simulink model "FinalSim"  (R2022b)
settings: Solver=VariableStepAuto  StartTime=0.0  StopTime=10  RelTol=1e-3
libraries: eeGeneralControl x3
(part 6 of 7)

== system FinalSim/Bicep Model/Bicep Group1/fascicles (CE & PE)/Type F Motor Units/Motor Unit 1 ==
  fenv : Inport
  Y,L : Inport  Port=2
  1/Tf (feff' < 0) : Fcn  Expr=u(2)/(0.02822+0.01513*u(3))
  1/Tf (feff' > 0) : Fcn  Expr=1/(0.02057*u(2)^2+0.0136*u(4))
  1/Ts : Gain  Gain=23.2558  SaturateOnIntegerOverflow=on  OutDataTypeStr=Inherit: Same as input  ParamDataTypeStr=Inherit: Same as input
  Af : Fcn  Expr=1-exp(-(u(1)*u(4)*u(3)/(0.56*u(2)))^u(2))
  Leff' : Fcn  Expr=(u(2)-u(1))^3/((1-u(3))*8.8e-005)
  Leff'->Leff : Integrator  InitialCondition=1
  "Leff,L, Af,fenv" : Mux
  S and old S diff : Sum  Inputs=-+  InputSameDT=on  SaturateOnIntegerOverflow=on  OutDataTypeStr=Inherit: Same as first input
  Y,nf,feff,S : Mux
  aS1 : Constant  Value=1.76
  aS2 : Constant  Value=0.96
  demux Y,L : Demux  Outputs=2
      settings: DisplayOption=none
  feff' : Product  InputSameDT=on  RndMeth=Zero  SaturateOnIntegerOverflow=on  OutDataTypeStr=Inherit: Same as first input
  feff' > 0? : Switch
  feff'->feff : Integrator
  feff>0.1? : Switch  Threshold=0.1
  fenv-fint : Sum  Inputs=+-  InputSameDT=on  SaturateOnIntegerOverflow=on  OutDataTypeStr=Inherit: Same as first input
  fint' : Product  InputSameDT=on  RndMeth=Zero  SaturateOnIntegerOverflow=on  OutDataTypeStr=Inherit: Same as first input
  fint'->fint : Integrator
  fint-feff : Sum  Inputs=+-  InputSameDT=on  SaturateOnIntegerOverflow=on  OutDataTypeStr=Inherit: Same as first input
  nf : Fcn  Expr=2.11+3.31*(1/u-1)
  s'->s : Integrator  InitialCondition=1.76
  A : Outport
  wires:
  Y,L/1 -> demux Y,L/1
  demux Y,L/1 -> Y,nf,feff,S/1
  demux Y,L/2 -> "Leff,L, Af,fenv"/2
  "Leff,L, Af,fenv"/1 -> 1/Tf (feff' < 0)/1, Leff'/1, 1/Tf (feff' > 0)/1
  1/Tf (feff' > 0)/1 -> feff' > 0?/1
  1/Tf (feff' < 0)/1 -> feff' > 0?/3
  fenv/1 -> fenv-fint/1, "Leff,L, Af,fenv"/4
  fenv-fint/1 -> fint'/2
  fint'/1 -> fint'->fint/1
  fint'->fint/1 -> fint-feff/1, fenv-fint/2
  fint-feff/1 -> feff'/2, feff' > 0?/2
  feff' > 0?/1 -> feff'/1, fint'/1
  feff'/1 -> feff'->feff/1
  feff'->feff/1 -> fint-feff/2, Y,nf,feff,S/3, feff>0.1?/2
  Y,nf,feff,S/1 -> Af/1
  Af/1 -> "Leff,L, Af,fenv"/3, A/1
  Leff'/1 -> Leff'->Leff/1
  Leff'->Leff/1 -> "Leff,L, Af,fenv"/1, nf/1
  nf/1 -> Y,nf,feff,S/2
  aS2/1 -> feff>0.1?/1
  aS1/1 -> feff>0.1?/3
  feff>0.1?/1 -> S and old S diff/2
  S and old S diff/1 -> 1/Ts/1
  1/Ts/1 -> s'->s/1
  s'->s/1 -> S and old S diff/1, Y,nf,feff,S/4

== system FinalSim/Bicep Model/Bicep Group1/fascicles (CE & PE)/Type F Motor Units/Motor Unit 2 ==
  fenv : Inport
  Y,L : Inport  Port=2
  1/Tf (feff' < 0) : Fcn  Expr=u(2)/(0.02822+0.01513*u(3))
  1/Tf (feff' > 0) : Fcn  Expr=1/(0.02057*u(2)^2+0.0136*u(4))
  1/Ts : Gain  Gain=23.2558  SaturateOnIntegerOverflow=on  OutDataTypeStr=Inherit: Same as input  ParamDataTypeStr=Inherit: Same as input
  Af : Fcn  Expr=1-exp(-(u(1)*u(4)*u(3)/(0.56*u(2)))^u(2))
  Leff' : Fcn  Expr=(u(2)-u(1))^3/((1-u(3))*8.8e-005)
  Leff'->Leff : Integrator  InitialCondition=1
  "Leff,L, Af,fenv" : Mux
  S and old S diff : Sum  Inputs=-+  InputSameDT=on  SaturateOnIntegerOverflow=on  OutDataTypeStr=Inherit: Same as first input
  Y,nf,feff,S : Mux
  aS1 : Constant  Value=1.76
  aS2 : Constant  Value=0.96
  demux Y,L : Demux  Outputs=2
      settings: DisplayOption=none
  feff' : Product  InputSameDT=on  RndMeth=Zero  SaturateOnIntegerOverflow=on  OutDataTypeStr=Inherit: Same as first input
  feff' > 0? : Switch
  feff'->feff : Integrator
  feff>0.1? : Switch  Threshold=0.1
  fenv-fint : Sum  Inputs=+-  InputSameDT=on  SaturateOnIntegerOverflow=on  OutDataTypeStr=Inherit: Same as first input
  fint' : Product  InputSameDT=on  RndMeth=Zero  SaturateOnIntegerOverflow=on  OutDataTypeStr=Inherit: Same as first input
  fint'->fint : Integrator
  fint-feff : Sum  Inputs=+-  InputSameDT=on  SaturateOnIntegerOverflow=on  OutDataTypeStr=Inherit: Same as first input
  nf : Fcn  Expr=2.11+3.31*(1/u-1)
  s'->s : Integrator  InitialCondition=1.76
  A : Outport
  wires:
  Y,L/1 -> demux Y,L/1
  demux Y,L/1 -> Y,nf,feff,S/1
  demux Y,L/2 -> "Leff,L, Af,fenv"/2
  "Leff,L, Af,fenv"/1 -> 1/Tf (feff' < 0)/1, Leff'/1, 1/Tf (feff' > 0)/1
  1/Tf (feff' > 0)/1 -> feff' > 0?/1
  1/Tf (feff' < 0)/1 -> feff' > 0?/3
  fenv/1 -> fenv-fint/1, "Leff,L, Af,fenv"/4
  fenv-fint/1 -> fint'/2
  fint'/1 -> fint'->fint/1
  fint'->fint/1 -> fint-feff/1, fenv-fint/2
  fint-feff/1 -> feff'/2, feff' > 0?/2
  feff' > 0?/1 -> feff'/1, fint'/1
  feff'/1 -> feff'->feff/1
  feff'->feff/1 -> fint-feff/2, Y,nf,feff,S/3, feff>0.1?/2
  Y,nf,feff,S/1 -> Af/1
  Af/1 -> "Leff,L, Af,fenv"/3, A/1
  Leff'/1 -> Leff'->Leff/1
  Leff'->Leff/1 -> "Leff,L, Af,fenv"/1, nf/1
  nf/1 -> Y,nf,feff,S/2
  aS2/1 -> feff>0.1?/1
  aS1/1 -> feff>0.1?/3
  feff>0.1?/1 -> S and old S diff/2
  S and old S diff/1 -> 1/Ts/1
  1/Ts/1 -> s'->s/1
  s'->s/1 -> S and old S diff/1, Y,nf,feff,S/4

== system FinalSim/Bicep Model/Bicep Group1/fascicles (CE & PE)/Type F Motor Units/Motor Unit 3 ==
  fenv : Inport
  Y,L : Inport  Port=2
  1/Tf (feff' < 0) : Fcn  Expr=u(2)/(0.02822+0.01513*u(3))
  1/Tf (feff' > 0) : Fcn  Expr=1/(0.02057*u(2)^2+0.0136*u(4))
  1/Ts : Gain  Gain=23.2558  SaturateOnIntegerOverflow=on  OutDataTypeStr=Inherit: Same as input  ParamDataTypeStr=Inherit: Same as input
  Af : Fcn  Expr=1-exp(-(u(1)*u(4)*u(3)/(0.56*u(2)))^u(2))
  Leff' : Fcn  Expr=(u(2)-u(1))^3/((1-u(3))*8.8e-005)
  Leff'->Leff : Integrator  InitialCondition=1
  "Leff,L, Af,fenv" : Mux
  S and old S diff : Sum  Inputs=-+  InputSameDT=on  SaturateOnIntegerOverflow=on  OutDataTypeStr=Inherit: Same as first input
  Y,nf,feff,S : Mux
  aS1 : Constant  Value=1.76
  aS2 : Constant  Value=0.96
  demux Y,L : Demux  Outputs=2
      settings: DisplayOption=none
  feff' : Product  InputSameDT=on  RndMeth=Zero  SaturateOnIntegerOverflow=on  OutDataTypeStr=Inherit: Same as first input
  feff' > 0? : Switch
  feff'->feff : Integrator
  feff>0.1? : Switch  Threshold=0.1
  fenv-fint : Sum  Inputs=+-  InputSameDT=on  SaturateOnIntegerOverflow=on  OutDataTypeStr=Inherit: Same as first input
  fint' : Product  InputSameDT=on  RndMeth=Zero  SaturateOnIntegerOverflow=on  OutDataTypeStr=Inherit: Same as first input
  fint'->fint : Integrator
  fint-feff : Sum  Inputs=+-  InputSameDT=on  SaturateOnIntegerOverflow=on  OutDataTypeStr=Inherit: Same as first input
  nf : Fcn  Expr=2.11+3.31*(1/u-1)
  s'->s : Integrator  InitialCondition=1.76
  A : Outport
  wires:
  Y,L/1 -> demux Y,L/1
  demux Y,L/1 -> Y,nf,feff,S/1
  demux Y,L/2 -> "Leff,L, Af,fenv"/2
  "Leff,L, Af,fenv"/1 -> 1/Tf (feff' < 0)/1, Leff'/1, 1/Tf (feff' > 0)/1
  1/Tf (feff' > 0)/1 -> feff' > 0?/1
  1/Tf (feff' < 0)/1 -> feff' > 0?/3
  fenv/1 -> fenv-fint/1, "Leff,L, Af,fenv"/4
  fenv-fint/1 -> fint'/2
  fint'/1 -> fint'->fint/1
  fint'->fint/1 -> fint-feff/1, fenv-fint/2
  fint-feff/1 -> feff'/2, feff' > 0?/2
  feff' > 0?/1 -> feff'/1, fint'/1
  feff'/1 -> feff'->feff/1
  feff'->feff/1 -> fint-feff/2, Y,nf,feff,S/3, feff>0.1?/2
  Y,nf,feff,S/1 -> Af/1
  Af/1 -> "Leff,L, Af,fenv"/3, A/1
  Leff'/1 -> Leff'->Leff/1
  Leff'->Leff/1 -> "Leff,L, Af,fenv"/1, nf/1
  nf/1 -> Y,nf,feff,S/2
  aS2/1 -> feff>0.1?/1
  aS1/1 -> feff>0.1?/3
  feff>0.1?/1 -> S and old S diff/2
  S and old S diff/1 -> 1/Ts/1
  1/Ts/1 -> s'->s/1
  s'->s/1 -> S and old S diff/1, Y,nf,feff,S/4

== system FinalSim/Bicep Model/Bicep Group1/fascicles (CE & PE)/Type S Motor Units/Motor Unit 1 ==
  fenv : Inport
  Y,L : Inport  Port=2
  1/Tf (feff' < 0) : Fcn  Expr=u(2)/(0.047033+0.025217*u(3))
  1/Tf (feff' > 0) : Fcn  Expr=1/(0.034283*u(2)^2+0.022667*u(4))
  Af : Fcn  Expr=1-exp(-(u(1)*u(4)*u(3)/(0.56*u(2)))^u(2))
  Leff' : Fcn  Expr=(u(2)-u(1))^3/((1-u(3))*8.8e-005)
  Leff'->Leff : Integrator  InitialCondition=1
  "Leff,L, Af,fenv" : Mux
  Y,nf,feff,S : Mux
  aS : Constant
  demux Y,L : Demux  Outputs=2
      settings: DisplayOption=none
  feff' : Product  InputSameDT=on  RndMeth=Zero  SaturateOnIntegerOverflow=on  OutDataTypeStr=Inherit: Same as first input
  feff' > 0? : Switch
  feff'->feff : Integrator
  fenv-fint : Sum  Inputs=+-  InputSameDT=on  SaturateOnIntegerOverflow=on  OutDataTypeStr=Inherit: Same as first input
  fint' : Product  InputSameDT=on  RndMeth=Zero  SaturateOnIntegerOverflow=on  OutDataTypeStr=Inherit: Same as first input
  fint'->fint : Integrator
  fint-feff : Sum  Inputs=+-  InputSameDT=on  SaturateOnIntegerOverflow=on  OutDataTypeStr=Inherit: Same as first input
  nf : Fcn  Expr=2.11+5*(1/u-1)
  A : Outport
  wires:
  Y,L/1 -> demux Y,L/1
  demux Y,L/1 -> Y,nf,feff,S/1
  demux Y,L/2 -> "Leff,L, Af,fenv"/2
  "Leff,L, Af,fenv"/1 -> 1/Tf (feff' < 0)/1, Leff'/1, 1/Tf (feff' > 0)/1
  1/Tf (feff' > 0)/1 -> feff' > 0?/1
  1/Tf (feff' < 0)/1 -> feff' > 0?/3
  fenv/1 -> fenv-fint/1, "Leff,L, Af,fenv"/4
  fenv-fint/1 -> fint'/2
  fint'/1 -> fint'->fint/1
  fint'->fint/1 -> fint-feff/1, fenv-fint/2
  fint-feff/1 -> feff'/2, feff' > 0?/2
  feff' > 0?/1 -> feff'/1, fint'/1
  feff'/1 -> feff'->feff/1
  feff'->feff/1 -> Y,nf,feff,S/3, fint-feff/2
  Y,nf,feff,S/1 -> Af/1
  Af/1 -> "Leff,L, Af,fenv"/3, A/1
  Leff'/1 -> Leff'->Leff/1
  Leff'->Leff/1 -> "Leff,L, Af,fenv"/1, nf/1
  nf/1 -> Y,nf,feff,S/2
  aS/1 -> Y,nf,feff,S/4

== system FinalSim/Bicep Model/Bicep Group1/fascicles (CE & PE)/Type S Motor Units/Motor Unit 2 ==
  fenv : Inport
  Y,L : Inport  Port=2
  1/Tf (feff' < 0) : Fcn  Expr=u(2)/(0.047033+0.025217*u(3))
  1/Tf (feff' > 0) : Fcn  Expr=1/(0.034283*u(2)^2+0.022667*u(4))
  Af : Fcn  Expr=1-exp(-(u(1)*u(4)*u(3)/(0.56*u(2)))^u(2))
  Leff' : Fcn  Expr=(u(2)-u(1))^3/((1-u(3))*8.8e-005)
  Leff'->Leff : Integrator  InitialCondition=1
  "Leff,L, Af,fenv" : Mux
  Y,nf,feff,S : Mux
  aS : Constant
  demux Y,L : Demux  Outputs=2
      settings: DisplayOption=none
  feff' : Product  InputSameDT=on  RndMeth=Zero  SaturateOnIntegerOverflow=on  OutDataTypeStr=Inherit: Same as first input
  feff' > 0? : Switch
  feff'->feff : Integrator
  fenv-fint : Sum  Inputs=+-  InputSameDT=on  SaturateOnIntegerOverflow=on  OutDataTypeStr=Inherit: Same as first input
  fint' : Product  InputSameDT=on  RndMeth=Zero  SaturateOnIntegerOverflow=on  OutDataTypeStr=Inherit: Same as first input
  fint'->fint : Integrator
  fint-feff : Sum  Inputs=+-  InputSameDT=on  SaturateOnIntegerOverflow=on  OutDataTypeStr=Inherit: Same as first input
  nf : Fcn  Expr=2.11+5*(1/u-1)
  A : Outport
  wires:
  Y,L/1 -> demux Y,L/1
  demux Y,L/1 -> Y,nf,feff,S/1
  demux Y,L/2 -> "Leff,L, Af,fenv"/2
  "Leff,L, Af,fenv"/1 -> 1/Tf (feff' < 0)/1, Leff'/1, 1/Tf (feff' > 0)/1
  1/Tf (feff' > 0)/1 -> feff' > 0?/1
  1/Tf (feff' < 0)/1 -> feff' > 0?/3
  fenv/1 -> fenv-fint/1, "Leff,L, Af,fenv"/4
  fenv-fint/1 -> fint'/2
  fint'/1 -> fint'->fint/1
  fint'->fint/1 -> fint-feff/1, fenv-fint/2
  fint-feff/1 -> feff'/2, feff' > 0?/2
  feff' > 0?/1 -> feff'/1, fint'/1
  feff'/1 -> feff'->feff/1
  feff'->feff/1 -> Y,nf,feff,S/3, fint-feff/2
  Y,nf,feff,S/1 -> Af/1
  Af/1 -> "Leff,L, Af,fenv"/3, A/1
  Leff'/1 -> Leff'->Leff/1
  Leff'->Leff/1 -> "Leff,L, Af,fenv"/1, nf/1
  nf/1 -> Y,nf,feff,S/2
  aS/1 -> Y,nf,feff,S/4

== system FinalSim/Shoulder Abductor Model/Shoulder Abductors1/fascicles (CE & PE)/Type F Motor Units/Motor Unit 1 ==
  fenv : Inport
  Y,L : Inport  Port=2
  1/Tf (feff' < 0) : Fcn  Expr=u(2)/(0.02822+0.01513*u(3))
  1/Tf (feff' > 0) : Fcn  Expr=1/(0.02057*u(2)^2+0.0136*u(4))
  1/Ts : Gain  Gain=23.2558  SaturateOnIntegerOverflow=on  OutDataTypeStr=Inherit: Same as input  ParamDataTypeStr=Inherit: Same as input
  Af : Fcn  Expr=1-exp(-(u(1)*u(4)*u(3)/(0.56*u(2)))^u(2))
  Leff' : Fcn  Expr=(u(2)-u(1))^3/((1-u(3))*8.8e-005)
  Leff'->Leff : Integrator  InitialCondition=1
  "Leff,L, Af,fenv" : Mux
  S and old S diff : Sum  Inputs=-+  InputSameDT=on  SaturateOnIntegerOverflow=on  OutDataTypeStr=Inherit: Same as first input
  Y,nf,feff,S : Mux
  aS1 : Constant  Value=1.76
  aS2 : Constant  Value=0.96
  demux Y,L : Demux  Outputs=2
      settings: DisplayOption=none
  feff' : Product  InputSameDT=on  RndMeth=Zero  SaturateOnIntegerOverflow=on  OutDataTypeStr=Inherit: Same as first input
  feff' > 0? : Switch
  feff'->feff : Integrator
  feff>0.1? : Switch  Threshold=0.1
  fenv-fint : Sum  Inputs=+-  InputSameDT=on  SaturateOnIntegerOverflow=on  OutDataTypeStr=Inherit: Same as first input
  fint' : Product  InputSameDT=on  RndMeth=Zero  SaturateOnIntegerOverflow=on  OutDataTypeStr=Inherit: Same as first input
  fint'->fint : Integrator
  fint-feff : Sum  Inputs=+-  InputSameDT=on  SaturateOnIntegerOverflow=on  OutDataTypeStr=Inherit: Same as first input
  nf : Fcn  Expr=2.11+3.31*(1/u-1)
  s'->s : Integrator  InitialCondition=1.76
  A : Outport
  wires:
  Y,L/1 -> demux Y,L/1
  demux Y,L/1 -> Y,nf,feff,S/1
  demux Y,L/2 -> "Leff,L, Af,fenv"/2
  "Leff,L, Af,fenv"/1 -> 1/Tf (feff' < 0)/1, Leff'/1, 1/Tf (feff' > 0)/1
  1/Tf (feff' > 0)/1 -> feff' > 0?/1
  1/Tf (feff' < 0)/1 -> feff' > 0?/3
  fenv/1 -> fenv-fint/1, "Leff,L, Af,fenv"/4
  fenv-fint/1 -> fint'/2
  fint'/1 -> fint'->fint/1
  fint'->fint/1 -> fint-feff/1, fenv-fint/2
  fint-feff/1 -> feff'/2, feff' > 0?/2
  feff' > 0?/1 -> feff'/1, fint'/1
  feff'/1 -> feff'->feff/1
  feff'->feff/1 -> fint-feff/2, Y,nf,feff,S/3, feff>0.1?/2
  Y,nf,feff,S/1 -> Af/1
  Af/1 -> "Leff,L, Af,fenv"/3, A/1
  Leff'/1 -> Leff'->Leff/1
  Leff'->Leff/1 -> "Leff,L, Af,fenv"/1, nf/1
  nf/1 -> Y,nf,feff,S/2
  aS2/1 -> feff>0.1?/1
  aS1/1 -> feff>0.1?/3
  feff>0.1?/1 -> S and old S diff/2
  S and old S diff/1 -> 1/Ts/1
  1/Ts/1 -> s'->s/1
  s'->s/1 -> S and old S diff/1, Y,nf,feff,S/4

== system FinalSim/Shoulder Abductor Model/Shoulder Abductors1/fascicles (CE & PE)/Type F Motor Units/Motor Unit 2 ==
  fenv : Inport
  Y,L : Inport  Port=2
  1/Tf (feff' < 0) : Fcn  Expr=u(2)/(0.02822+0.01513*u(3))
  1/Tf (feff' > 0) : Fcn  Expr=1/(0.02057*u(2)^2+0.0136*u(4))
  1/Ts : Gain  Gain=23.2558  SaturateOnIntegerOverflow=on  OutDataTypeStr=Inherit: Same as input  ParamDataTypeStr=Inherit: Same as input
  Af : Fcn  Expr=1-exp(-(u(1)*u(4)*u(3)/(0.56*u(2)))^u(2))
  Leff' : Fcn  Expr=(u(2)-u(1))^3/((1-u(3))*8.8e-005)
  Leff'->Leff : Integrator  InitialCondition=1
  "Leff,L, Af,fenv" : Mux
  S and old S diff : Sum  Inputs=-+  InputSameDT=on  SaturateOnIntegerOverflow=on  OutDataTypeStr=Inherit: Same as first input
  Y,nf,feff,S : Mux
  aS1 : Constant  Value=1.76
  aS2 : Constant  Value=0.96
  demux Y,L : Demux  Outputs=2
      settings: DisplayOption=none
  feff' : Product  InputSameDT=on  RndMeth=Zero  SaturateOnIntegerOverflow=on  OutDataTypeStr=Inherit: Same as first input
  feff' > 0? : Switch
  feff'->feff : Integrator
  feff>0.1? : Switch  Threshold=0.1
  fenv-fint : Sum  Inputs=+-  InputSameDT=on  SaturateOnIntegerOverflow=on  OutDataTypeStr=Inherit: Same as first input
  fint' : Product  InputSameDT=on  RndMeth=Zero  SaturateOnIntegerOverflow=on  OutDataTypeStr=Inherit: Same as first input
  fint'->fint : Integrator
  fint-feff : Sum  Inputs=+-  InputSameDT=on  SaturateOnIntegerOverflow=on  OutDataTypeStr=Inherit: Same as first input
  nf : Fcn  Expr=2.11+3.31*(1/u-1)
  s'->s : Integrator  InitialCondition=1.76
  A : Outport
  wires:
  Y,L/1 -> demux Y,L/1
  demux Y,L/1 -> Y,nf,feff,S/1
  demux Y,L/2 -> "Leff,L, Af,fenv"/2
  "Leff,L, Af,fenv"/1 -> 1/Tf (feff' < 0)/1, Leff'/1, 1/Tf (feff' > 0)/1
  1/Tf (feff' > 0)/1 -> feff' > 0?/1
  1/Tf (feff' < 0)/1 -> feff' > 0?/3
  fenv/1 -> fenv-fint/1, "Leff,L, Af,fenv"/4
  fenv-fint/1 -> fint'/2
  fint'/1 -> fint'->fint/1
  fint'->fint/1 -> fint-feff/1, fenv-fint/2
  fint-feff/1 -> feff'/2, feff' > 0?/2
  feff' > 0?/1 -> feff'/1, fint'/1
  feff'/1 -> feff'->feff/1
  feff'->feff/1 -> fint-feff/2, Y,nf,feff,S/3, feff>0.1?/2
  Y,nf,feff,S/1 -> Af/1
  Af/1 -> "Leff,L, Af,fenv"/3, A/1
  Leff'/1 -> Leff'->Leff/1
  Leff'->Leff/1 -> "Leff,L, Af,fenv"/1, nf/1
  nf/1 -> Y,nf,feff,S/2
  aS2/1 -> feff>0.1?/1
  aS1/1 -> feff>0.1?/3
  feff>0.1?/1 -> S and old S diff/2
  S and old S diff/1 -> 1/Ts/1
  1/Ts/1 -> s'->s/1
  s'->s/1 -> S and old S diff/1, Y,nf,feff,S/4

== system FinalSim/Shoulder Abductor Model/Shoulder Abductors1/fascicles (CE & PE)/Type F Motor Units/Motor Unit 3 ==
  fenv : Inport
  Y,L : Inport  Port=2
  1/Tf (feff' < 0) : Fcn  Expr=u(2)/(0.02822+0.01513*u(3))
  1/Tf (feff' > 0) : Fcn  Expr=1/(0.02057*u(2)^2+0.0136*u(4))
  1/Ts : Gain  Gain=23.2558  SaturateOnIntegerOverflow=on  OutDataTypeStr=Inherit: Same as input  ParamDataTypeStr=Inherit: Same as input
  Af : Fcn  Expr=1-exp(-(u(1)*u(4)*u(3)/(0.56*u(2)))^u(2))
  Leff' : Fcn  Expr=(u(2)-u(1))^3/((1-u(3))*8.8e-005)
  Leff'->Leff : Integrator  InitialCondition=1
  "Leff,L, Af,fenv" : Mux
  S and old S diff : Sum  Inputs=-+  InputSameDT=on  SaturateOnIntegerOverflow=on  OutDataTypeStr=Inherit: Same as first input
  Y,nf,feff,S : Mux
  aS1 : Constant  Value=1.76
  aS2 : Constant  Value=0.96
  demux Y,L : Demux  Outputs=2
      settings: DisplayOption=none
  feff' : Product  InputSameDT=on  RndMeth=Zero  SaturateOnIntegerOverflow=on  OutDataTypeStr=Inherit: Same as first input
  feff' > 0? : Switch
  feff'->feff : Integrator
  feff>0.1? : Switch  Threshold=0.1
  fenv-fint : Sum  Inputs=+-  InputSameDT=on  SaturateOnIntegerOverflow=on  OutDataTypeStr=Inherit: Same as first input
  fint' : Product  InputSameDT=on  RndMeth=Zero  SaturateOnIntegerOverflow=on  OutDataTypeStr=Inherit: Same as first input
  fint'->fint : Integrator
  fint-feff : Sum  Inputs=+-  InputSameDT=on  SaturateOnIntegerOverflow=on  OutDataTypeStr=Inherit: Same as first input
  nf : Fcn  Expr=2.11+3.31*(1/u-1)
  s'->s : Integrator  InitialCondition=1.76
  A : Outport
  wires:
  Y,L/1 -> demux Y,L/1
  demux Y,L/1 -> Y,nf,feff,S/1
  demux Y,L/2 -> "Leff,L, Af,fenv"/2
  "Leff,L, Af,fenv"/1 -> 1/Tf (feff' < 0)/1, Leff'/1, 1/Tf (feff' > 0)/1
  1/Tf (feff' > 0)/1 -> feff' > 0?/1
  1/Tf (feff' < 0)/1 -> feff' > 0?/3
  fenv/1 -> fenv-fint/1, "Leff,L, Af,fenv"/4
  fenv-fint/1 -> fint'/2
  fint'/1 -> fint'->fint/1
  fint'->fint/1 -> fint-feff/1, fenv-fint/2
  fint-feff/1 -> feff'/2, feff' > 0?/2
  feff' > 0?/1 -> feff'/1, fint'/1
  feff'/1 -> feff'->feff/1
  feff'->feff/1 -> fint-feff/2, Y,nf,feff,S/3, feff>0.1?/2
  Y,nf,feff,S/1 -> Af/1
  Af/1 -> "Leff,L, Af,fenv"/3, A/1
  Leff'/1 -> Leff'->Leff/1
  Leff'->Leff/1 -> "Leff,L, Af,fenv"/1, nf/1
  nf/1 -> Y,nf,feff,S/2
  aS2/1 -> feff>0.1?/1
  aS1/1 -> feff>0.1?/3
  feff>0.1?/1 -> S and old S diff/2
  S and old S diff/1 -> 1/Ts/1
  1/Ts/1 -> s'->s/1
  s'->s/1 -> S and old S diff/1, Y,nf,feff,S/4

== system FinalSim/Shoulder Abductor Model/Shoulder Abductors1/fascicles (CE & PE)/Type S Motor Units/Motor Unit 1 ==
  fenv : Inport
  Y,L : Inport  Port=2
  1/Tf (feff' < 0) : Fcn  Expr=u(2)/(0.047033+0.025217*u(3))
  1/Tf (feff' > 0) : Fcn  Expr=1/(0.034283*u(2)^2+0.022667*u(4))
  Af : Fcn  Expr=1-exp(-(u(1)*u(4)*u(3)/(0.56*u(2)))^u(2))
  Leff' : Fcn  Expr=(u(2)-u(1))^3/((1-u(3))*8.8e-005)
  Leff'->Leff : Integrator  InitialCondition=1
  "Leff,L, Af,fenv" : Mux
  Y,nf,feff,S : Mux
  aS : Constant
  demux Y,L : Demux  Outputs=2
      settings: DisplayOption=none
  feff' : Product  InputSameDT=on  RndMeth=Zero  SaturateOnIntegerOverflow=on  OutDataTypeStr=Inherit: Same as first input
  feff' > 0? : Switch
  feff'->feff : Integrator
  fenv-fint : Sum  Inputs=+-  InputSameDT=on  SaturateOnIntegerOverflow=on  OutDataTypeStr=Inherit: Same as first input
  fint' : Product  InputSameDT=on  RndMeth=Zero  SaturateOnIntegerOverflow=on  OutDataTypeStr=Inherit: Same as first input
  fint'->fint : Integrator
  fint-feff : Sum  Inputs=+-  InputSameDT=on  SaturateOnIntegerOverflow=on  OutDataTypeStr=Inherit: Same as first input
  nf : Fcn  Expr=2.11+5*(1/u-1)
  A : Outport
  wires:
  Y,L/1 -> demux Y,L/1
  demux Y,L/1 -> Y,nf,feff,S/1
  demux Y,L/2 -> "Leff,L, Af,fenv"/2
  "Leff,L, Af,fenv"/1 -> 1/Tf (feff' < 0)/1, Leff'/1, 1/Tf (feff' > 0)/1
  1/Tf (feff' > 0)/1 -> feff' > 0?/1
  1/Tf (feff' < 0)/1 -> feff' > 0?/3
  fenv/1 -> fenv-fint/1, "Leff,L, Af,fenv"/4
  fenv-fint/1 -> fint'/2
  fint'/1 -> fint'->fint/1
  fint'->fint/1 -> fint-feff/1, fenv-fint/2
  fint-feff/1 -> feff'/2, feff' > 0?/2
  feff' > 0?/1 -> feff'/1, fint'/1
  feff'/1 -> feff'->feff/1
  feff'->feff/1 -> Y,nf,feff,S/3, fint-feff/2
  Y,nf,feff,S/1 -> Af/1
  Af/1 -> "Leff,L, Af,fenv"/3, A/1
  Leff'/1 -> Leff'->Leff/1
  Leff'->Leff/1 -> "Leff,L, Af,fenv"/1, nf/1
  nf/1 -> Y,nf,feff,S/2
  aS/1 -> Y,nf,feff,S/4

== system FinalSim/Shoulder Abductor Model/Shoulder Abductors1/fascicles (CE & PE)/Type S Motor Units/Motor Unit 2 ==
  fenv : Inport
  Y,L : Inport  Port=2
  1/Tf (feff' < 0) : Fcn  Expr=u(2)/(0.047033+0.025217*u(3))
  1/Tf (feff' > 0) : Fcn  Expr=1/(0.034283*u(2)^2+0.022667*u(4))
  Af : Fcn  Expr=1-exp(-(u(1)*u(4)*u(3)/(0.56*u(2)))^u(2))
  Leff' : Fcn  Expr=(u(2)-u(1))^3/((1-u(3))*8.8e-005)
  Leff'->Leff : Integrator  InitialCondition=1
  "Leff,L, Af,fenv" : Mux
  Y,nf,feff,S : Mux
  aS : Constant
  demux Y,L : Demux  Outputs=2
      settings: DisplayOption=none
  feff' : Product  InputSameDT=on  RndMeth=Zero  SaturateOnIntegerOverflow=on  OutDataTypeStr=Inherit: Same as first input
  feff' > 0? : Switch
  feff'->feff : Integrator
  fenv-fint : Sum  Inputs=+-  InputSameDT=on  SaturateOnIntegerOverflow=on  OutDataTypeStr=Inherit: Same as first input
  fint' : Product  InputSameDT=on  RndMeth=Zero  SaturateOnIntegerOverflow=on  OutDataTypeStr=Inherit: Same as first input
  fint'->fint : Integrator
  fint-feff : Sum  Inputs=+-  InputSameDT=on  SaturateOnIntegerOverflow=on  OutDataTypeStr=Inherit: Same as first input
  nf : Fcn  Expr=2.11+5*(1/u-1)
  A : Outport
  wires:
  Y,L/1 -> demux Y,L/1
  demux Y,L/1 -> Y,nf,feff,S/1
  demux Y,L/2 -> "Leff,L, Af,fenv"/2
  "Leff,L, Af,fenv"/1 -> 1/Tf (feff' < 0)/1, Leff'/1, 1/Tf (feff' > 0)/1
  1/Tf (feff' > 0)/1 -> feff' > 0?/1
  1/Tf (feff' < 0)/1 -> feff' > 0?/3
  fenv/1 -> fenv-fint/1, "Leff,L, Af,fenv"/4
  fenv-fint/1 -> fint'/2
  fint'/1 -> fint'->fint/1
  fint'->fint/1 -> fint-feff/1, fenv-fint/2
  fint-feff/1 -> feff'/2, feff' > 0?/2
  feff' > 0?/1 -> feff'/1, fint'/1
  feff'/1 -> feff'->feff/1
  feff'->feff/1 -> Y,nf,feff,S/3, fint-feff/2
  Y,nf,feff,S/1 -> Af/1
  Af/1 -> "Leff,L, Af,fenv"/3, A/1
  Leff'/1 -> Leff'->Leff/1
  Leff'->Leff/1 -> "Leff,L, Af,fenv"/1, nf/1
  nf/1 -> Y,nf,feff,S/2
  aS/1 -> Y,nf,feff,S/4

== system FinalSim/Shoulder Adductor Model/Shoulder Transverse Flexors1/fascicles (CE & PE)/Type F Motor Units/Motor Unit 1 ==
  fenv : Inport
  Y,L : Inport  Port=2
  1/Tf (feff' < 0) : Fcn  Expr=u(2)/(0.02822+0.01513*u(3))
  1/Tf (feff' > 0) : Fcn  Expr=1/(0.02057*u(2)^2+0.0136*u(4))
  1/Ts : Gain  Gain=23.2558  SaturateOnIntegerOverflow=on  OutDataTypeStr=Inherit: Same as input  ParamDataTypeStr=Inherit: Same as input
  Af : Fcn  Expr=1-exp(-(u(1)*u(4)*u(3)/(0.56*u(2)))^u(2))
  Leff' : Fcn  Expr=(u(2)-u(1))^3/((1-u(3))*8.8e-005)
  Leff'->Leff : Integrator  InitialCondition=1
  "Leff,L, Af,fenv" : Mux
  S and old S diff : Sum  Inputs=-+  InputSameDT=on  SaturateOnIntegerOverflow=on  OutDataTypeStr=Inherit: Same as first input
  Y,nf,feff,S : Mux
  aS1 : Constant  Value=1.76
  aS2 : Constant  Value=0.96
  demux Y,L : Demux  Outputs=2
      settings: DisplayOption=none
  feff' : Product  InputSameDT=on  RndMeth=Zero  SaturateOnIntegerOverflow=on  OutDataTypeStr=Inherit: Same as first input
  feff' > 0? : Switch
  feff'->feff : Integrator
  feff>0.1? : Switch  Threshold=0.1
  fenv-fint : Sum  Inputs=+-  InputSameDT=on  SaturateOnIntegerOverflow=on  OutDataTypeStr=Inherit: Same as first input
  fint' : Product  InputSameDT=on  RndMeth=Zero  SaturateOnIntegerOverflow=on  OutDataTypeStr=Inherit: Same as first input
  fint'->fint : Integrator
  fint-feff : Sum  Inputs=+-  InputSameDT=on  SaturateOnIntegerOverflow=on  OutDataTypeStr=Inherit: Same as first input
  nf : Fcn  Expr=2.11+3.31*(1/u-1)
  s'->s : Integrator  InitialCondition=1.76
  A : Outport
  wires:
  Y,L/1 -> demux Y,L/1
  demux Y,L/1 -> Y,nf,feff,S/1
  demux Y,L/2 -> "Leff,L, Af,fenv"/2
  "Leff,L, Af,fenv"/1 -> 1/Tf (feff' < 0)/1, Leff'/1, 1/Tf (feff' > 0)/1
  1/Tf (feff' > 0)/1 -> feff' > 0?/1
  1/Tf (feff' < 0)/1 -> feff' > 0?/3
  fenv/1 -> fenv-fint/1, "Leff,L, Af,fenv"/4
  fenv-fint/1 -> fint'/2
  fint'/1 -> fint'->fint/1
  fint'->fint/1 -> fint-feff/1, fenv-fint/2
  fint-feff/1 -> feff'/2, feff' > 0?/2
  feff' > 0?/1 -> feff'/1, fint'/1
  feff'/1 -> feff'->feff/1
  feff'->feff/1 -> fint-feff/2, Y,nf,feff,S/3, feff>0.1?/2
  Y,nf,feff,S/1 -> Af/1
  Af/1 -> "Leff,L, Af,fenv"/3, A/1
  Leff'/1 -> Leff'->Leff/1
  Leff'->Leff/1 -> "Leff,L, Af,fenv"/1, nf/1
  nf/1 -> Y,nf,feff,S/2
  aS2/1 -> feff>0.1?/1
  aS1/1 -> feff>0.1?/3
  feff>0.1?/1 -> S and old S diff/2
  S and old S diff/1 -> 1/Ts/1
  1/Ts/1 -> s'->s/1
  s'->s/1 -> S and old S diff/1, Y,nf,feff,S/4

== system FinalSim/Shoulder Adductor Model/Shoulder Transverse Flexors1/fascicles (CE & PE)/Type F Motor Units/Motor Unit 2 ==
  fenv : Inport
  Y,L : Inport  Port=2
  1/Tf (feff' < 0) : Fcn  Expr=u(2)/(0.02822+0.01513*u(3))
  1/Tf (feff' > 0) : Fcn  Expr=1/(0.02057*u(2)^2+0.0136*u(4))
  1/Ts : Gain  Gain=23.2558  SaturateOnIntegerOverflow=on  OutDataTypeStr=Inherit: Same as input  ParamDataTypeStr=Inherit: Same as input
  Af : Fcn  Expr=1-exp(-(u(1)*u(4)*u(3)/(0.56*u(2)))^u(2))
  Leff' : Fcn  Expr=(u(2)-u(1))^3/((1-u(3))*8.8e-005)
  Leff'->Leff : Integrator  InitialCondition=1
  "Leff,L, Af,fenv" : Mux
  S and old S diff : Sum  Inputs=-+  InputSameDT=on  SaturateOnIntegerOverflow=on  OutDataTypeStr=Inherit: Same as first input
  Y,nf,feff,S : Mux
  aS1 : Constant  Value=1.76
  aS2 : Constant  Value=0.96
  demux Y,L : Demux  Outputs=2
      settings: DisplayOption=none
  feff' : Product  InputSameDT=on  RndMeth=Zero  SaturateOnIntegerOverflow=on  OutDataTypeStr=Inherit: Same as first input
  feff' > 0? : Switch
  feff'->feff : Integrator
  feff>0.1? : Switch  Threshold=0.1
  fenv-fint : Sum  Inputs=+-  InputSameDT=on  SaturateOnIntegerOverflow=on  OutDataTypeStr=Inherit: Same as first input
  fint' : Product  InputSameDT=on  RndMeth=Zero  SaturateOnIntegerOverflow=on  OutDataTypeStr=Inherit: Same as first input
  fint'->fint : Integrator
  fint-feff : Sum  Inputs=+-  InputSameDT=on  SaturateOnIntegerOverflow=on  OutDataTypeStr=Inherit: Same as first input
  nf : Fcn  Expr=2.11+3.31*(1/u-1)
  s'->s : Integrator  InitialCondition=1.76
  A : Outport
  wires:
  Y,L/1 -> demux Y,L/1
  demux Y,L/1 -> Y,nf,feff,S/1
  demux Y,L/2 -> "Leff,L, Af,fenv"/2
  "Leff,L, Af,fenv"/1 -> 1/Tf (feff' < 0)/1, Leff'/1, 1/Tf (feff' > 0)/1
  1/Tf (feff' > 0)/1 -> feff' > 0?/1
  1/Tf (feff' < 0)/1 -> feff' > 0?/3
  fenv/1 -> fenv-fint/1, "Leff,L, Af,fenv"/4
  fenv-fint/1 -> fint'/2
  fint'/1 -> fint'->fint/1
  fint'->fint/1 -> fint-feff/1, fenv-fint/2
  fint-feff/1 -> feff'/2, feff' > 0?/2
  feff' > 0?/1 -> feff'/1, fint'/1
  feff'/1 -> feff'->feff/1
  feff'->feff/1 -> fint-feff/2, Y,nf,feff,S/3, feff>0.1?/2
  Y,nf,feff,S/1 -> Af/1
  Af/1 -> "Leff,L, Af,fenv"/3, A/1
  Leff'/1 -> Leff'->Leff/1
  Leff'->Leff/1 -> "Leff,L, Af,fenv"/1, nf/1
  nf/1 -> Y,nf,feff,S/2
  aS2/1 -> feff>0.1?/1
  aS1/1 -> feff>0.1?/3
  feff>0.1?/1 -> S and old S diff/2
  S and old S diff/1 -> 1/Ts/1
  1/Ts/1 -> s'->s/1
  s'->s/1 -> S and old S diff/1, Y,nf,feff,S/4

== system FinalSim/Shoulder Adductor Model/Shoulder Transverse Flexors1/fascicles (CE & PE)/Type F Motor Units/Motor Unit 3 ==
  fenv : Inport
  Y,L : Inport  Port=2
  1/Tf (feff' < 0) : Fcn  Expr=u(2)/(0.02822+0.01513*u(3))
  1/Tf (feff' > 0) : Fcn  Expr=1/(0.02057*u(2)^2+0.0136*u(4))
  1/Ts : Gain  Gain=23.2558  SaturateOnIntegerOverflow=on  OutDataTypeStr=Inherit: Same as input  ParamDataTypeStr=Inherit: Same as input
  Af : Fcn  Expr=1-exp(-(u(1)*u(4)*u(3)/(0.56*u(2)))^u(2))
  Leff' : Fcn  Expr=(u(2)-u(1))^3/((1-u(3))*8.8e-005)
  Leff'->Leff : Integrator  InitialCondition=1
  "Leff,L, Af,fenv" : Mux
  S and old S diff : Sum  Inputs=-+  InputSameDT=on  SaturateOnIntegerOverflow=on  OutDataTypeStr=Inherit: Same as first input
  Y,nf,feff,S : Mux
  aS1 : Constant  Value=1.76
  aS2 : Constant  Value=0.96
  demux Y,L : Demux  Outputs=2
      settings: DisplayOption=none
  feff' : Product  InputSameDT=on  RndMeth=Zero  SaturateOnIntegerOverflow=on  OutDataTypeStr=Inherit: Same as first input
  feff' > 0? : Switch
  feff'->feff : Integrator
  feff>0.1? : Switch  Threshold=0.1
  fenv-fint : Sum  Inputs=+-  InputSameDT=on  SaturateOnIntegerOverflow=on  OutDataTypeStr=Inherit: Same as first input
  fint' : Product  InputSameDT=on  RndMeth=Zero  SaturateOnIntegerOverflow=on  OutDataTypeStr=Inherit: Same as first input
  fint'->fint : Integrator
  fint-feff : Sum  Inputs=+-  InputSameDT=on  SaturateOnIntegerOverflow=on  OutDataTypeStr=Inherit: Same as first input
  nf : Fcn  Expr=2.11+3.31*(1/u-1)
  s'->s : Integrator  InitialCondition=1.76
  A : Outport
  wires:
  Y,L/1 -> demux Y,L/1
  demux Y,L/1 -> Y,nf,feff,S/1
  demux Y,L/2 -> "Leff,L, Af,fenv"/2
  "Leff,L, Af,fenv"/1 -> 1/Tf (feff' < 0)/1, Leff'/1, 1/Tf (feff' > 0)/1
  1/Tf (feff' > 0)/1 -> feff' > 0?/1
  1/Tf (feff' < 0)/1 -> feff' > 0?/3
  fenv/1 -> fenv-fint/1, "Leff,L, Af,fenv"/4
  fenv-fint/1 -> fint'/2
  fint'/1 -> fint'->fint/1
  fint'->fint/1 -> fint-feff/1, fenv-fint/2
  fint-feff/1 -> feff'/2, feff' > 0?/2
  feff' > 0?/1 -> feff'/1, fint'/1
  feff'/1 -> feff'->feff/1
  feff'->feff/1 -> fint-feff/2, Y,nf,feff,S/3, feff>0.1?/2
  Y,nf,feff,S/1 -> Af/1
  Af/1 -> "Leff,L, Af,fenv"/3, A/1
  Leff'/1 -> Leff'->Leff/1
  Leff'->Leff/1 -> "Leff,L, Af,fenv"/1, nf/1
  nf/1 -> Y,nf,feff,S/2
  aS2/1 -> feff>0.1?/1
  aS1/1 -> feff>0.1?/3
  feff>0.1?/1 -> S and old S diff/2
  S and old S diff/1 -> 1/Ts/1
  1/Ts/1 -> s'->s/1
  s'->s/1 -> S and old S diff/1, Y,nf,feff,S/4

== system FinalSim/Shoulder Adductor Model/Shoulder Transverse Flexors1/fascicles (CE & PE)/Type S Motor Units/Motor Unit 1 ==
  fenv : Inport
  Y,L : Inport  Port=2
  1/Tf (feff' < 0) : Fcn  Expr=u(2)/(0.047033+0.025217*u(3))
  1/Tf (feff' > 0) : Fcn  Expr=1/(0.034283*u(2)^2+0.022667*u(4))
  Af : Fcn  Expr=1-exp(-(u(1)*u(4)*u(3)/(0.56*u(2)))^u(2))
  Leff' : Fcn  Expr=(u(2)-u(1))^3/((1-u(3))*8.8e-005)
  Leff'->Leff : Integrator  InitialCondition=1
  "Leff,L, Af,fenv" : Mux
  Y,nf,feff,S : Mux
  aS : Constant
  demux Y,L : Demux  Outputs=2
      settings: DisplayOption=none
  feff' : Product  InputSameDT=on  RndMeth=Zero  SaturateOnIntegerOverflow=on  OutDataTypeStr=Inherit: Same as first input
  feff' > 0? : Switch
  feff'->feff : Integrator
  fenv-fint : Sum  Inputs=+-  InputSameDT=on  SaturateOnIntegerOverflow=on  OutDataTypeStr=Inherit: Same as first input
  fint' : Product  InputSameDT=on  RndMeth=Zero  SaturateOnIntegerOverflow=on  OutDataTypeStr=Inherit: Same as first input
  fint'->fint : Integrator
  fint-feff : Sum  Inputs=+-  InputSameDT=on  SaturateOnIntegerOverflow=on  OutDataTypeStr=Inherit: Same as first input
  nf : Fcn  Expr=2.11+5*(1/u-1)
  A : Outport
  wires:
  Y,L/1 -> demux Y,L/1
  demux Y,L/1 -> Y,nf,feff,S/1
  demux Y,L/2 -> "Leff,L, Af,fenv"/2
  "Leff,L, Af,fenv"/1 -> 1/Tf (feff' < 0)/1, Leff'/1, 1/Tf (feff' > 0)/1
  1/Tf (feff' > 0)/1 -> feff' > 0?/1
  1/Tf (feff' < 0)/1 -> feff' > 0?/3
  fenv/1 -> fenv-fint/1, "Leff,L, Af,fenv"/4
  fenv-fint/1 -> fint'/2
  fint'/1 -> fint'->fint/1
  fint'->fint/1 -> fint-feff/1, fenv-fint/2
  fint-feff/1 -> feff'/2, feff' > 0?/2
  feff' > 0?/1 -> feff'/1, fint'/1
  feff'/1 -> feff'->feff/1
  feff'->feff/1 -> Y,nf,feff,S/3, fint-feff/2
  Y,nf,feff,S/1 -> Af/1
  Af/1 -> "Leff,L, Af,fenv"/3, A/1
  Leff'/1 -> Leff'->Leff/1
  Leff'->Leff/1 -> "Leff,L, Af,fenv"/1, nf/1
  nf/1 -> Y,nf,feff,S/2
  aS/1 -> Y,nf,feff,S/4

== system FinalSim/Shoulder Adductor Model/Shoulder Transverse Flexors1/fascicles (CE & PE)/Type S Motor Units/Motor Unit 2 ==
  fenv : Inport
  Y,L : Inport  Port=2
  1/Tf (feff' < 0) : Fcn  Expr=u(2)/(0.047033+0.025217*u(3))
  1/Tf (feff' > 0) : Fcn  Expr=1/(0.034283*u(2)^2+0.022667*u(4))
  Af : Fcn  Expr=1-exp(-(u(1)*u(4)*u(3)/(0.56*u(2)))^u(2))
  Leff' : Fcn  Expr=(u(2)-u(1))^3/((1-u(3))*8.8e-005)
  Leff'->Leff : Integrator  InitialCondition=1
  "Leff,L, Af,fenv" : Mux
  Y,nf,feff,S : Mux
  aS : Constant
  demux Y,L : Demux  Outputs=2
      settings: DisplayOption=none
  feff' : Product  InputSameDT=on  RndMeth=Zero  SaturateOnIntegerOverflow=on  OutDataTypeStr=Inherit: Same as first input
  feff' > 0? : Switch
  feff'->feff : Integrator
  fenv-fint : Sum  Inputs=+-  InputSameDT=on  SaturateOnIntegerOverflow=on  OutDataTypeStr=Inherit: Same as first input
  fint' : Product  InputSameDT=on  RndMeth=Zero  SaturateOnIntegerOverflow=on  OutDataTypeStr=Inherit: Same as first input
  fint'->fint : Integrator
  fint-feff : Sum  Inputs=+-  InputSameDT=on  SaturateOnIntegerOverflow=on  OutDataTypeStr=Inherit: Same as first input
  nf : Fcn  Expr=2.11+5*(1/u-1)
  A : Outport
  wires:
  Y,L/1 -> demux Y,L/1
  demux Y,L/1 -> Y,nf,feff,S/1
  demux Y,L/2 -> "Leff,L, Af,fenv"/2
  "Leff,L, Af,fenv"/1 -> 1/Tf (feff' < 0)/1, Leff'/1, 1/Tf (feff' > 0)/1
  1/Tf (feff' > 0)/1 -> feff' > 0?/1
  1/Tf (feff' < 0)/1 -> feff' > 0?/3
  fenv/1 -> fenv-fint/1, "Leff,L, Af,fenv"/4
  fenv-fint/1 -> fint'/2
  fint'/1 -> fint'->fint/1
  fint'->fint/1 -> fint-feff/1, fenv-fint/2
  fint-feff/1 -> feff'/2, feff' > 0?/2
  feff' > 0?/1 -> feff'/1, fint'/1
  feff'/1 -> feff'->feff/1
  feff'->feff/1 -> Y,nf,feff,S/3, fint-feff/2
  Y,nf,feff,S/1 -> Af/1
  Af/1 -> "Leff,L, Af,fenv"/3, A/1
  Leff'/1 -> Leff'->Leff/1
  Leff'->Leff/1 -> "Leff,L, Af,fenv"/1, nf/1
  nf/1 -> Y,nf,feff,S/2
  aS/1 -> Y,nf,feff,S/4

== system FinalSim/Shoulder Extensor Model/Shoulder Abductors1/fascicles (CE & PE)/Type F Motor Units/Motor Unit 1 ==
  fenv : Inport
  Y,L : Inport  Port=2
  1/Tf (feff' < 0) : Fcn  Expr=u(2)/(0.02822+0.01513*u(3))
  1/Tf (feff' > 0) : Fcn  Expr=1/(0.02057*u(2)^2+0.0136*u(4))
  1/Ts : Gain  Gain=23.2558  SaturateOnIntegerOverflow=on  OutDataTypeStr=Inherit: Same as input  ParamDataTypeStr=Inherit: Same as input
  Af : Fcn  Expr=1-exp(-(u(1)*u(4)*u(3)/(0.56*u(2)))^u(2))
  Leff' : Fcn  Expr=(u(2)-u(1))^3/((1-u(3))*8.8e-005)
  Leff'->Leff : Integrator  InitialCondition=1
  "Leff,L, Af,fenv" : Mux
  S and old S diff : Sum  Inputs=-+  InputSameDT=on  SaturateOnIntegerOverflow=on  OutDataTypeStr=Inherit: Same as first input
  Y,nf,feff,S : Mux
  aS1 : Constant  Value=1.76
  aS2 : Constant  Value=0.96
  demux Y,L : Demux  Outputs=2
      settings: DisplayOption=none
  feff' : Product  InputSameDT=on  RndMeth=Zero  SaturateOnIntegerOverflow=on  OutDataTypeStr=Inherit: Same as first input
  feff' > 0? : Switch
  feff'->feff : Integrator
  feff>0.1? : Switch  Threshold=0.1
  fenv-fint : Sum  Inputs=+-  InputSameDT=on  SaturateOnIntegerOverflow=on  OutDataTypeStr=Inherit: Same as first input
  fint' : Product  InputSameDT=on  RndMeth=Zero  SaturateOnIntegerOverflow=on  OutDataTypeStr=Inherit: Same as first input
  fint'->fint : Integrator
  fint-feff : Sum  Inputs=+-  InputSameDT=on  SaturateOnIntegerOverflow=on  OutDataTypeStr=Inherit: Same as first input
  nf : Fcn  Expr=2.11+3.31*(1/u-1)
  s'->s : Integrator  InitialCondition=1.76
  A : Outport
  wires:
  Y,L/1 -> demux Y,L/1
  demux Y,L/1 -> Y,nf,feff,S/1
  demux Y,L/2 -> "Leff,L, Af,fenv"/2
  "Leff,L, Af,fenv"/1 -> 1/Tf (feff' < 0)/1, Leff'/1, 1/Tf (feff' > 0)/1
  1/Tf (feff' > 0)/1 -> feff' > 0?/1
  1/Tf (feff' < 0)/1 -> feff' > 0?/3
  fenv/1 -> fenv-fint/1, "Leff,L, Af,fenv"/4
  fenv-fint/1 -> fint'/2
  fint'/1 -> fint'->fint/1
  fint'->fint/1 -> fint-feff/1, fenv-fint/2
  fint-feff/1 -> feff'/2, feff' > 0?/2
  feff' > 0?/1 -> feff'/1, fint'/1
  feff'/1 -> feff'->feff/1
  feff'->feff/1 -> fint-feff/2, Y,nf,feff,S/3, feff>0.1?/2
  Y,nf,feff,S/1 -> Af/1
  Af/1 -> "Leff,L, Af,fenv"/3, A/1
  Leff'/1 -> Leff'->Leff/1
  Leff'->Leff/1 -> "Leff,L, Af,fenv"/1, nf/1
  nf/1 -> Y,nf,feff,S/2
  aS2/1 -> feff>0.1?/1
  aS1/1 -> feff>0.1?/3
  feff>0.1?/1 -> S and old S diff/2
  S and old S diff/1 -> 1/Ts/1
  1/Ts/1 -> s'->s/1
  s'->s/1 -> S and old S diff/1, Y,nf,feff,S/4

== system FinalSim/Shoulder Extensor Model/Shoulder Abductors1/fascicles (CE & PE)/Type F Motor Units/Motor Unit 2 ==
  fenv : Inport
  Y,L : Inport  Port=2
  1/Tf (feff' < 0) : Fcn  Expr=u(2)/(0.02822+0.01513*u(3))
  1/Tf (feff' > 0) : Fcn  Expr=1/(0.02057*u(2)^2+0.0136*u(4))
  1/Ts : Gain  Gain=23.2558  SaturateOnIntegerOverflow=on  OutDataTypeStr=Inherit: Same as input  ParamDataTypeStr=Inherit: Same as input
  Af : Fcn  Expr=1-exp(-(u(1)*u(4)*u(3)/(0.56*u(2)))^u(2))
  Leff' : Fcn  Expr=(u(2)-u(1))^3/((1-u(3))*8.8e-005)
  Leff'->Leff : Integrator  InitialCondition=1
  "Leff,L, Af,fenv" : Mux
  S and old S diff : Sum  Inputs=-+  InputSameDT=on  SaturateOnIntegerOverflow=on  OutDataTypeStr=Inherit: Same as first input
  Y,nf,feff,S : Mux
  aS1 : Constant  Value=1.76
  aS2 : Constant  Value=0.96
  demux Y,L : Demux  Outputs=2
      settings: DisplayOption=none
  feff' : Product  InputSameDT=on  RndMeth=Zero  SaturateOnIntegerOverflow=on  OutDataTypeStr=Inherit: Same as first input
  feff' > 0? : Switch
  feff'->feff : Integrator
  feff>0.1? : Switch  Threshold=0.1
  fenv-fint : Sum  Inputs=+-  InputSameDT=on  SaturateOnIntegerOverflow=on  OutDataTypeStr=Inherit: Same as first input
  fint' : Product  InputSameDT=on  RndMeth=Zero  SaturateOnIntegerOverflow=on  OutDataTypeStr=Inherit: Same as first input
  fint'->fint : Integrator
  fint-feff : Sum  Inputs=+-  InputSameDT=on  SaturateOnIntegerOverflow=on  OutDataTypeStr=Inherit: Same as first input
  nf : Fcn  Expr=2.11+3.31*(1/u-1)
  s'->s : Integrator  InitialCondition=1.76
  A : Outport
  wires:
  Y,L/1 -> demux Y,L/1
  demux Y,L/1 -> Y,nf,feff,S/1
  demux Y,L/2 -> "Leff,L, Af,fenv"/2
  "Leff,L, Af,fenv"/1 -> 1/Tf (feff' < 0)/1, Leff'/1, 1/Tf (feff' > 0)/1
  1/Tf (feff' > 0)/1 -> feff' > 0?/1
  1/Tf (feff' < 0)/1 -> feff' > 0?/3
  fenv/1 -> fenv-fint/1, "Leff,L, Af,fenv"/4
  fenv-fint/1 -> fint'/2
  fint'/1 -> fint'->fint/1
  fint'->fint/1 -> fint-feff/1, fenv-fint/2
  fint-feff/1 -> feff'/2, feff' > 0?/2
  feff' > 0?/1 -> feff'/1, fint'/1
  feff'/1 -> feff'->feff/1
  feff'->feff/1 -> fint-feff/2, Y,nf,feff,S/3, feff>0.1?/2
  Y,nf,feff,S/1 -> Af/1
  Af/1 -> "Leff,L, Af,fenv"/3, A/1
  Leff'/1 -> Leff'->Leff/1
  Leff'->Leff/1 -> "Leff,L, Af,fenv"/1, nf/1
  nf/1 -> Y,nf,feff,S/2
  aS2/1 -> feff>0.1?/1
  aS1/1 -> feff>0.1?/3
  feff>0.1?/1 -> S and old S diff/2
  S and old S diff/1 -> 1/Ts/1
  1/Ts/1 -> s'->s/1
  s'->s/1 -> S and old S diff/1, Y,nf,feff,S/4

== system FinalSim/Shoulder Extensor Model/Shoulder Abductors1/fascicles (CE & PE)/Type F Motor Units/Motor Unit 3 ==
  fenv : Inport
  Y,L : Inport  Port=2
  1/Tf (feff' < 0) : Fcn  Expr=u(2)/(0.02822+0.01513*u(3))
  1/Tf (feff' > 0) : Fcn  Expr=1/(0.02057*u(2)^2+0.0136*u(4))
  1/Ts : Gain  Gain=23.2558  SaturateOnIntegerOverflow=on  OutDataTypeStr=Inherit: Same as input  ParamDataTypeStr=Inherit: Same as input
  Af : Fcn  Expr=1-exp(-(u(1)*u(4)*u(3)/(0.56*u(2)))^u(2))
  Leff' : Fcn  Expr=(u(2)-u(1))^3/((1-u(3))*8.8e-005)
  Leff'->Leff : Integrator  InitialCondition=1
  "Leff,L, Af,fenv" : Mux
  S and old S diff : Sum  Inputs=-+  InputSameDT=on  SaturateOnIntegerOverflow=on  OutDataTypeStr=Inherit: Same as first input
  Y,nf,feff,S : Mux
  aS1 : Constant  Value=1.76
  aS2 : Constant  Value=0.96
  demux Y,L : Demux  Outputs=2
      settings: DisplayOption=none
  feff' : Product  InputSameDT=on  RndMeth=Zero  SaturateOnIntegerOverflow=on  OutDataTypeStr=Inherit: Same as first input
  feff' > 0? : Switch
  feff'->feff : Integrator
  feff>0.1? : Switch  Threshold=0.1
  fenv-fint : Sum  Inputs=+-  InputSameDT=on  SaturateOnIntegerOverflow=on  OutDataTypeStr=Inherit: Same as first input
  fint' : Product  InputSameDT=on  RndMeth=Zero  SaturateOnIntegerOverflow=on  OutDataTypeStr=Inherit: Same as first input
  fint'->fint : Integrator
  fint-feff : Sum  Inputs=+-  InputSameDT=on  SaturateOnIntegerOverflow=on  OutDataTypeStr=Inherit: Same as first input
  nf : Fcn  Expr=2.11+3.31*(1/u-1)
  s'->s : Integrator  InitialCondition=1.76
  A : Outport
  wires:
  Y,L/1 -> demux Y,L/1
  demux Y,L/1 -> Y,nf,feff,S/1
  demux Y,L/2 -> "Leff,L, Af,fenv"/2
  "Leff,L, Af,fenv"/1 -> 1/Tf (feff' < 0)/1, Leff'/1, 1/Tf (feff' > 0)/1
  1/Tf (feff' > 0)/1 -> feff' > 0?/1
  1/Tf (feff' < 0)/1 -> feff' > 0?/3
  fenv/1 -> fenv-fint/1, "Leff,L, Af,fenv"/4
  fenv-fint/1 -> fint'/2
  fint'/1 -> fint'->fint/1
  fint'->fint/1 -> fint-feff/1, fenv-fint/2
  fint-feff/1 -> feff'/2, feff' > 0?/2
  feff' > 0?/1 -> feff'/1, fint'/1
  feff'/1 -> feff'->feff/1
  feff'->feff/1 -> fint-feff/2, Y,nf,feff,S/3, feff>0.1?/2
  Y,nf,feff,S/1 -> Af/1
  Af/1 -> "Leff,L, Af,fenv"/3, A/1
  Leff'/1 -> Leff'->Leff/1
  Leff'->Leff/1 -> "Leff,L, Af,fenv"/1, nf/1
  nf/1 -> Y,nf,feff,S/2
  aS2/1 -> feff>0.1?/1
  aS1/1 -> feff>0.1?/3
  feff>0.1?/1 -> S and old S diff/2
  S and old S diff/1 -> 1/Ts/1
  1/Ts/1 -> s'->s/1
  s'->s/1 -> S and old S diff/1, Y,nf,feff,S/4

== system FinalSim/Shoulder Extensor Model/Shoulder Abductors1/fascicles (CE & PE)/Type S Motor Units/Motor Unit 1 ==
  fenv : Inport
  Y,L : Inport  Port=2
  1/Tf (feff' < 0) : Fcn  Expr=u(2)/(0.047033+0.025217*u(3))
  1/Tf (feff' > 0) : Fcn  Expr=1/(0.034283*u(2)^2+0.022667*u(4))
  Af : Fcn  Expr=1-exp(-(u(1)*u(4)*u(3)/(0.56*u(2)))^u(2))
  Leff' : Fcn  Expr=(u(2)-u(1))^3/((1-u(3))*8.8e-005)
  Leff'->Leff : Integrator  InitialCondition=1
  "Leff,L, Af,fenv" : Mux
  Y,nf,feff,S : Mux
  aS : Constant
  demux Y,L : Demux  Outputs=2
      settings: DisplayOption=none
  feff' : Product  InputSameDT=on  RndMeth=Zero  SaturateOnIntegerOverflow=on  OutDataTypeStr=Inherit: Same as first input
  feff' > 0? : Switch
  feff'->feff : Integrator
  fenv-fint : Sum  Inputs=+-  InputSameDT=on  SaturateOnIntegerOverflow=on  OutDataTypeStr=Inherit: Same as first input
  fint' : Product  InputSameDT=on  RndMeth=Zero  SaturateOnIntegerOverflow=on  OutDataTypeStr=Inherit: Same as first input
  fint'->fint : Integrator
  fint-feff : Sum  Inputs=+-  InputSameDT=on  SaturateOnIntegerOverflow=on  OutDataTypeStr=Inherit: Same as first input
  nf : Fcn  Expr=2.11+5*(1/u-1)
  A : Outport
  wires:
  Y,L/1 -> demux Y,L/1
  demux Y,L/1 -> Y,nf,feff,S/1
  demux Y,L/2 -> "Leff,L, Af,fenv"/2
  "Leff,L, Af,fenv"/1 -> 1/Tf (feff' < 0)/1, Leff'/1, 1/Tf (feff' > 0)/1
  1/Tf (feff' > 0)/1 -> feff' > 0?/1
  1/Tf (feff' < 0)/1 -> feff' > 0?/3
  fenv/1 -> fenv-fint/1, "Leff,L, Af,fenv"/4
  fenv-fint/1 -> fint'/2
  fint'/1 -> fint'->fint/1
  fint'->fint/1 -> fint-feff/1, fenv-fint/2
  fint-feff/1 -> feff'/2, feff' > 0?/2
  feff' > 0?/1 -> feff'/1, fint'/1
  feff'/1 -> feff'->feff/1
  feff'->feff/1 -> Y,nf,feff,S/3, fint-feff/2
  Y,nf,feff,S/1 -> Af/1
  Af/1 -> "Leff,L, Af,fenv"/3, A/1
  Leff'/1 -> Leff'->Leff/1
  Leff'->Leff/1 -> "Leff,L, Af,fenv"/1, nf/1
  nf/1 -> Y,nf,feff,S/2
  aS/1 -> Y,nf,feff,S/4

== system FinalSim/Shoulder Extensor Model/Shoulder Abductors1/fascicles (CE & PE)/Type S Motor Units/Motor Unit 2 ==
  fenv : Inport
  Y,L : Inport  Port=2
  1/Tf (feff' < 0) : Fcn  Expr=u(2)/(0.047033+0.025217*u(3))
  1/Tf (feff' > 0) : Fcn  Expr=1/(0.034283*u(2)^2+0.022667*u(4))
  Af : Fcn  Expr=1-exp(-(u(1)*u(4)*u(3)/(0.56*u(2)))^u(2))
  Leff' : Fcn  Expr=(u(2)-u(1))^3/((1-u(3))*8.8e-005)
  Leff'->Leff : Integrator  InitialCondition=1
  "Leff,L, Af,fenv" : Mux
  Y,nf,feff,S : Mux
  aS : Constant
  demux Y,L : Demux  Outputs=2
      settings: DisplayOption=none
  feff' : Product  InputSameDT=on  RndMeth=Zero  SaturateOnIntegerOverflow=on  OutDataTypeStr=Inherit: Same as first input
  feff' > 0? : Switch
  feff'->feff : Integrator
  fenv-fint : Sum  Inputs=+-  InputSameDT=on  SaturateOnIntegerOverflow=on  OutDataTypeStr=Inherit: Same as first input
  fint' : Product  InputSameDT=on  RndMeth=Zero  SaturateOnIntegerOverflow=on  OutDataTypeStr=Inherit: Same as first input
  fint'->fint : Integrator
  fint-feff : Sum  Inputs=+-  InputSameDT=on  SaturateOnIntegerOverflow=on  OutDataTypeStr=Inherit: Same as first input
  nf : Fcn  Expr=2.11+5*(1/u-1)
  A : Outport
  wires:
  Y,L/1 -> demux Y,L/1
  demux Y,L/1 -> Y,nf,feff,S/1
  demux Y,L/2 -> "Leff,L, Af,fenv"/2
  "Leff,L, Af,fenv"/1 -> 1/Tf (feff' < 0)/1, Leff'/1, 1/Tf (feff' > 0)/1
  1/Tf (feff' > 0)/1 -> feff' > 0?/1
  1/Tf (feff' < 0)/1 -> feff' > 0?/3
  fenv/1 -> fenv-fint/1, "Leff,L, Af,fenv"/4
  fenv-fint/1 -> fint'/2
  fint'/1 -> fint'->fint/1
  fint'->fint/1 -> fint-feff/1, fenv-fint/2
  fint-feff/1 -> feff'/2, feff' > 0?/2
  feff' > 0?/1 -> feff'/1, fint'/1
  feff'/1 -> feff'->feff/1
  feff'->feff/1 -> Y,nf,feff,S/3, fint-feff/2
  Y,nf,feff,S/1 -> Af/1
  Af/1 -> "Leff,L, Af,fenv"/3, A/1
  Leff'/1 -> Leff'->Leff/1
  Leff'->Leff/1 -> "Leff,L, Af,fenv"/1, nf/1
  nf/1 -> Y,nf,feff,S/2
  aS/1 -> Y,nf,feff,S/4

== system FinalSim/Shoulder Transverse Model/Shoulder Transverse Flexors1/fascicles (CE & PE)/Type F Motor Units/Motor Unit 1 ==
  fenv : Inport
  Y,L : Inport  Port=2
  1/Tf (feff' < 0) : Fcn  Expr=u(2)/(0.02822+0.01513*u(3))
  1/Tf (feff' > 0) : Fcn  Expr=1/(0.02057*u(2)^2+0.0136*u(4))
  1/Ts : Gain  Gain=23.2558  SaturateOnIntegerOverflow=on  OutDataTypeStr=Inherit: Same as input  ParamDataTypeStr=Inherit: Same as input
  Af : Fcn  Expr=1-exp(-(u(1)*u(4)*u(3)/(0.56*u(2)))^u(2))
  Leff' : Fcn  Expr=(u(2)-u(1))^3/((1-u(3))*8.8e-005)
  Leff'->Leff : Integrator  InitialCondition=1
  "Leff,L, Af,fenv" : Mux
  S and old S diff : Sum  Inputs=-+  InputSameDT=on  SaturateOnIntegerOverflow=on  OutDataTypeStr=Inherit: Same as first input
  Y,nf,feff,S : Mux
  aS1 : Constant  Value=1.76
  aS2 : Constant  Value=0.96
  demux Y,L : Demux  Outputs=2
      settings: DisplayOption=none
  feff' : Product  InputSameDT=on  RndMeth=Zero  SaturateOnIntegerOverflow=on  OutDataTypeStr=Inherit: Same as first input
  feff' > 0? : Switch
  feff'->feff : Integrator
  feff>0.1? : Switch  Threshold=0.1
  fenv-fint : Sum  Inputs=+-  InputSameDT=on  SaturateOnIntegerOverflow=on  OutDataTypeStr=Inherit: Same as first input
  fint' : Product  InputSameDT=on  RndMeth=Zero  SaturateOnIntegerOverflow=on  OutDataTypeStr=Inherit: Same as first input
  fint'->fint : Integrator
  fint-feff : Sum  Inputs=+-  InputSameDT=on  SaturateOnIntegerOverflow=on  OutDataTypeStr=Inherit: Same as first input
  nf : Fcn  Expr=2.11+3.31*(1/u-1)
  s'->s : Integrator  InitialCondition=1.76
  A : Outport
  wires:
  Y,L/1 -> demux Y,L/1
  demux Y,L/1 -> Y,nf,feff,S/1
  demux Y,L/2 -> "Leff,L, Af,fenv"/2
  "Leff,L, Af,fenv"/1 -> 1/Tf (feff' < 0)/1, Leff'/1, 1/Tf (feff' > 0)/1
  1/Tf (feff' > 0)/1 -> feff' > 0?/1
  1/Tf (feff' < 0)/1 -> feff' > 0?/3
  fenv/1 -> fenv-fint/1, "Leff,L, Af,fenv"/4
  fenv-fint/1 -> fint'/2
  fint'/1 -> fint'->fint/1
  fint'->fint/1 -> fint-feff/1, fenv-fint/2
  fint-feff/1 -> feff'/2, feff' > 0?/2
  feff' > 0?/1 -> feff'/1, fint'/1
  feff'/1 -> feff'->feff/1
  feff'->feff/1 -> fint-feff/2, Y,nf,feff,S/3, feff>0.1?/2
  Y,nf,feff,S/1 -> Af/1
  Af/1 -> "Leff,L, Af,fenv"/3, A/1
  Leff'/1 -> Leff'->Leff/1
  Leff'->Leff/1 -> "Leff,L, Af,fenv"/1, nf/1
  nf/1 -> Y,nf,feff,S/2
  aS2/1 -> feff>0.1?/1
  aS1/1 -> feff>0.1?/3
  feff>0.1?/1 -> S and old S diff/2
  S and old S diff/1 -> 1/Ts/1
  1/Ts/1 -> s'->s/1
  s'->s/1 -> S and old S diff/1, Y,nf,feff,S/4

== system FinalSim/Shoulder Transverse Model/Shoulder Transverse Flexors1/fascicles (CE & PE)/Type F Motor Units/Motor Unit 2 ==
  fenv : Inport
  Y,L : Inport  Port=2
  1/Tf (feff' < 0) : Fcn  Expr=u(2)/(0.02822+0.01513*u(3))
  1/Tf (feff' > 0) : Fcn  Expr=1/(0.02057*u(2)^2+0.0136*u(4))
  1/Ts : Gain  Gain=23.2558  SaturateOnIntegerOverflow=on  OutDataTypeStr=Inherit: Same as input  ParamDataTypeStr=Inherit: Same as input
  Af : Fcn  Expr=1-exp(-(u(1)*u(4)*u(3)/(0.56*u(2)))^u(2))
  Leff' : Fcn  Expr=(u(2)-u(1))^3/((1-u(3))*8.8e-005)
  Leff'->Leff : Integrator  InitialCondition=1
  "Leff,L, Af,fenv" : Mux
  S and old S diff : Sum  Inputs=-+  InputSameDT=on  SaturateOnIntegerOverflow=on  OutDataTypeStr=Inherit: Same as first input
  Y,nf,feff,S : Mux
  aS1 : Constant  Value=1.76
  aS2 : Constant  Value=0.96
  demux Y,L : Demux  Outputs=2
      settings: DisplayOption=none
  feff' : Product  InputSameDT=on  RndMeth=Zero  SaturateOnIntegerOverflow=on  OutDataTypeStr=Inherit: Same as first input
  feff' > 0? : Switch
  feff'->feff : Integrator
  feff>0.1? : Switch  Threshold=0.1
  fenv-fint : Sum  Inputs=+-  InputSameDT=on  SaturateOnIntegerOverflow=on  OutDataTypeStr=Inherit: Same as first input
  fint' : Product  InputSameDT=on  RndMeth=Zero  SaturateOnIntegerOverflow=on  OutDataTypeStr=Inherit: Same as first input
  fint'->fint : Integrator
  fint-feff : Sum  Inputs=+-  InputSameDT=on  SaturateOnIntegerOverflow=on  OutDataTypeStr=Inherit: Same as first input
  nf : Fcn  Expr=2.11+3.31*(1/u-1)
  s'->s : Integrator  InitialCondition=1.76
  A : Outport
  wires:
  Y,L/1 -> demux Y,L/1
  demux Y,L/1 -> Y,nf,feff,S/1
  demux Y,L/2 -> "Leff,L, Af,fenv"/2
  "Leff,L, Af,fenv"/1 -> 1/Tf (feff' < 0)/1, Leff'/1, 1/Tf (feff' > 0)/1
  1/Tf (feff' > 0)/1 -> feff' > 0?/1
  1/Tf (feff' < 0)/1 -> feff' > 0?/3
  fenv/1 -> fenv-fint/1, "Leff,L, Af,fenv"/4
  fenv-fint/1 -> fint'/2
  fint'/1 -> fint'->fint/1
  fint'->fint/1 -> fint-feff/1, fenv-fint/2
  fint-feff/1 -> feff'/2, feff' > 0?/2
  feff' > 0?/1 -> feff'/1, fint'/1
  feff'/1 -> feff'->feff/1
  feff'->feff/1 -> fint-feff/2, Y,nf,feff,S/3, feff>0.1?/2
  Y,nf,feff,S/1 -> Af/1
  Af/1 -> "Leff,L, Af,fenv"/3, A/1
  Leff'/1 -> Leff'->Leff/1
  Leff'->Leff/1 -> "Leff,L, Af,fenv"/1, nf/1
  nf/1 -> Y,nf,feff,S/2
  aS2/1 -> feff>0.1?/1
  aS1/1 -> feff>0.1?/3
  feff>0.1?/1 -> S and old S diff/2
  S and old S diff/1 -> 1/Ts/1
  1/Ts/1 -> s'->s/1
  s'->s/1 -> S and old S diff/1, Y,nf,feff,S/4
